simulink model "sampleModel1910"  (R2023a)
settings: Solver=VariableStepAuto  StartTime=0.0  StopTime=10.0  RelTol=1e-3
libraries: hdlsllib x3, simulink x1
settings Model: Creator=user1  LastModifiedBy=user1

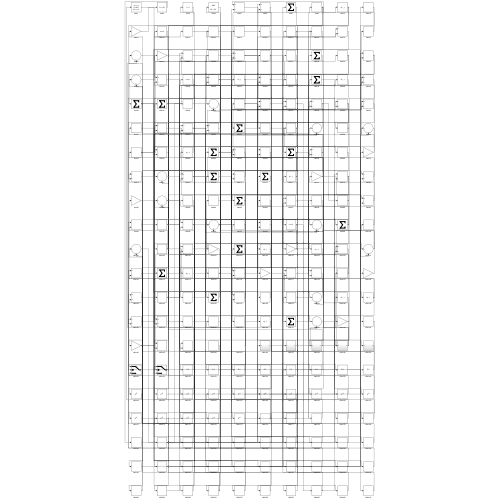
[thumbnail: Simulink's stored preview of the top-level diagram]
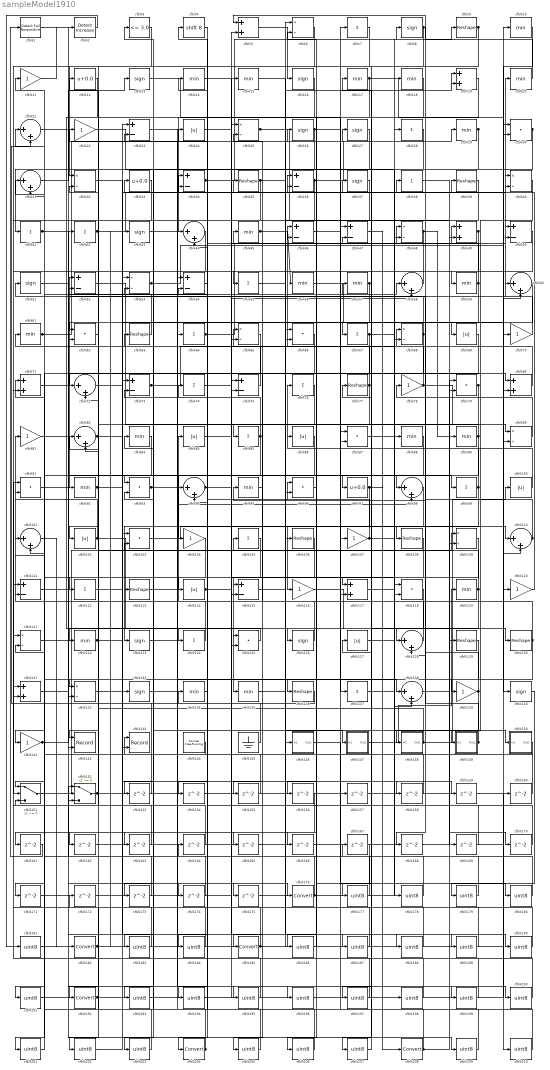
== system sampleModel1910 ==
  cfblk1 : hdlsllib/Logic and Bit Operations/Detect Fall Nonpositive  vinit=0  OutDataTypeStr=boolean
  cfblk{10,14..15,17..18,20,29,45,56..57,59,61,83,88..89,92,95,119,122,134..135} (21 alike) : MinMax
  cfblk{24,69,84,86,100,102,114,127} (8 alike) : Abs  SaturateOnIntegerOverflow=off
  cfblk{21,31,44,58,60,72,82,94,98,101,110,128,138} (13 alike) : Sum  Inputs=|++
  cfblk{30,62,66,79,87,91,93,96,103,118,125} (11 alike) : DotProduct  OutDataTypeStr=Inherit: Inherit via internal rule
  cfblk{11,22,70,78,81,104,107,116,120,139,141} (11 alike) : Gain
  cfblk{7,28,38,41..42,55,64,67,74,76,85,99,105,112,124,137} (16 alike) : Sum  Inputs=+
  cfblk{9,35,39,63,77,106,108,113,129..130,136} (11 alike) : Reshape
  cfblk{6,25,32,40,48,53,65,68,90,109,121,132} (12 alike) : Product  Inputs=*/  RndMeth=Zero  SaturateOnIntegerOverflow=on
  cfblk{23,34,36,46..47,50,52,54,73,75,111,115} (12 alike) : Sum  Inputs=+-
  cfblk{5,19,49,71,80,117,131} (7 alike) : Sum
  cfblk12 : Bias  Bias=0.0  SaturateOnIntegerOverflow=off
  cfblk{8,13,16,26..27,37,43,51,123,126,133,140} (12 alike) : Signum
  cfblk142 : Record  FileSettingsInternal="{\"entries\":[{\"content\":{\"excelSettings\":{\"content\":{},\"type\":\"Streamout.ExcelSettings\"}},\"type\":\"Streamout.FileSettingStorage\",\"uuid\":\"\"}],\"packageUris\":[\"http:\\/\\/schema.mathworks.com\\/mf0\\/streamout_blocks\\/R2020a\"],\"version\":\"1.0\"}"  Layout=[1 1]  SignalsInternal="{\"entries\":[{\"content\":{\"signals\":[{\"content\":{\"blockPath\":[],\"dimensions\":[1],\"domain\":\"\",\"lineColor\":\"#a2142f\",\"plots\":[1],\"port\":1,\"signalID\":5086,\"signalName\":\"XY Graph:1\"},\"type\":\"RecordBlkView.Signal\",\"uuid\":\"\"},{\"content\":{\"blockPath\":[],\"dimensions\":[1],\"domain\":\"\",\"lineColor\":\"#139fff\",\"plots\":[1],\"port\":2,\"signalID\":5089,\"signalName\":\"XY Graph:2\"},\"type\":\"RecordBlkView.Signal\",\"uuid\":\"\"}]},\"type\":\"RecordBlkView.InputSignals\",\"uuid\":\"\"}],\"packageUris\":[\"http:\\/\\/schema.mathworks.com\\/mf0\\/streamout_blocks\\/R2020a\"],\"version\":\"1.0\"}"  VisualizationBindings="{\"xyplotplugin\":{\"info\":[{\"series\":[{\"bindingParametersList\":[{\"parameter\":\"X-Axis\",\"signalID\":5086,\"signalName\":\"XY Graph:1\"},{\"parameter\":\"Y-Axis\",\"signalID\":5089,\"signalName\":\"XY Graph:2\"}],\"seriesID\":15448}],\"subplotID\":1}]}}"  CompatibilityTag=XY  st=-1
  cfblk143 : Record  FileSettingsInternal="{\"entries\":[{\"content\":{\"excelSettings\":{\"content\":{},\"type\":\"Streamout.ExcelSettings\"}},\"type\":\"Streamout.FileSettingStorage\",\"uuid\":\"\"}],\"packageUris\":[\"http:\\/\\/schema.mathworks.com\\/mf0\\/streamout_blocks\\/R2020a\"],\"version\":\"1.0\"}"  Layout=[1 1]  SignalsInternal="{\"entries\":[{\"content\":{\"signals\":[{\"content\":{\"blockPath\":[],\"dimensions\":[1],\"domain\":\"\",\"lineColor\":\"#a2142f\",\"plots\":[1],\"port\":1,\"signalID\":5094,\"signalName\":\"XY Graph:1\"},\"type\":\"RecordBlkView.Signal\",\"uuid\":\"\"},{\"content\":{\"blockPath\":[],\"dimensions\":[1],\"domain\":\"\",\"lineColor\":\"#139fff\",\"plots\":[1],\"port\":2,\"signalID\":5097,\"signalName\":\"XY Graph:2\"},\"type\":\"RecordBlkView.Signal\",\"uuid\":\"\"}]},\"type\":\"RecordBlkView.InputSignals\",\"uuid\":\"\"}],\"packageUris\":[\"http:\\/\\/schema.mathworks.com\\/mf0\\/streamout_blocks\\/R2020a\"],\"version\":\"1.0\"}"  VisualizationBindings="{\"xyplotplugin\":{\"info\":[{\"series\":[{\"bindingParametersList\":[{\"parameter\":\"X-Axis\",\"signalID\":5094,\"signalName\":\"XY Graph:1\"},{\"parameter\":\"Y-Axis\",\"signalID\":5097,\"signalName\":\"XY Graph:2\"}],\"seriesID\":38158}],\"subplotID\":1}]}}"  CompatibilityTag=XY  st=-1
  cfblk144 : hdlsllib/Sources/Counter Free-Running  NumBits=16  tsamp=-1
  cfblk145 : Ground
  cfblk146 : Subsystem
      settings: LibrarySourceBlock=|
      | hdlsllib/Ports &
      | Subsystems/Subsystem
  cfblk147 : Subsystem
      settings: LibrarySourceBlock=|
      | hdlsllib/Ports &
      | Subsystems/Subsystem
  cfblk148 : Subsystem
      settings: LibrarySourceBlock=|
      | hdlsllib/Ports &
      | Subsystems/Subsystem
  cfblk149 : Subsystem
      settings: LibrarySourceBlock=|
      | hdlsllib/Ports &
      | Subsystems/Subsystem
  cfblk150 : Subsystem
      settings: LibrarySourceBlock=|
      | hdlsllib/Ports &
      | Subsystems/Subsystem
  cfblk151 : Switch  SaturateOnIntegerOverflow=off  InputSameDT=off
  cfblk152 : Switch  SaturateOnIntegerOverflow=off  InputSameDT=off
  cfblk{153..175} (23 alike) : Delay  SampleTime=1
  cfblk{176,182,185,192,204,208} (6 alike) : DataTypeConversion  SaturateOnIntegerOverflow=off  RndMeth=Floor
  cfblk{177..181,183..184,186..191,193..203,205..207,209..210} (29 alike) : DataTypeConversion  OutDataTypeStr=uint8  SaturateOnIntegerOverflow=off  RndMeth=Floor
  cfblk2 : simulink/Logic and Bit Operations/Detect Increase  vinit=0.0  OutDataTypeStr=boolean
      settings: LibrarySourceBlock=|
      | hdlsllib/Logic and Bit
      | Operations/Detect
      | Increase
  cfblk3 : hdlsllib/Logic and Bit Operations/Compare To Constant  relop=<=  const=3.0  OutDataTypeStr=boolean
  cfblk33 : Bias  Bias=0.0  SaturateOnIntegerOverflow=off
  cfblk4 : ArithShift  BitShiftNumber=8
  cfblk97 : Bias  Bias=0.0  SaturateOnIntegerOverflow=off
  wires:
  cfblk65/1 -> cfblk92/1
  cfblk64/1 -> cfblk48/1, cfblk36/2
  cfblk148/1(Out1) -> cfblk100/1, cfblk52/2
  cfblk77/1 -> cfblk46/1, cfblk94/2
  cfblk120/1 -> cfblk33/1
  cfblk115/1 -> cfblk6/1
  cfblk5/1 -> cfblk16/1
  cfblk58/1 -> cfblk55/1
  cfblk16/1 -> cfblk44/1
  cfblk12/1 -> cfblk126/1
  cfblk150/1(Out1) -> cfblk84/1
  cfblk61/1 -> cfblk24/1, cfblk60/1
  cfblk48/1 -> cfblk89/1, cfblk72/1
  cfblk131/1 -> cfblk42/1
  cfblk6/1 -> cfblk32/1
  cfblk116/1 -> cfblk128/1
  cfblk128/1 -> cfblk81/1
  cfblk98/1 -> cfblk116/1
  cfblk104/1 -> cfblk114/1
  cfblk52/1 -> cfblk90/1
  cfblk99/1 -> cfblk123/1, cfblk77/1, cfblk94/1
  cfblk11/1 -> cfblk2/1
  cfblk114/1 -> cfblk74/1, cfblk188/1
  cfblk79/1 -> cfblk102/1, cfblk148/1(In1)
  cfblk50/1 -> cfblk59/1
  cfblk97/1 -> cfblk173/1, cfblk198/1
  cfblk25/1 -> cfblk107/1, cfblk19/2, cfblk49/2
  cfblk136/1 -> cfblk21/2
  cfblk151/1 -> cfblk64/1
  cfblk28/1 -> cfblk41/1
  cfblk102/1 -> cfblk130/1, cfblk71/1
  cfblk34/1 -> cfblk8/1, cfblk58/2
  cfblk113/1 -> cfblk138/1
  cfblk27/1 -> cfblk113/1
  cfblk72/1 -> cfblk133/1
  cfblk85/1 -> cfblk3/1, cfblk104/1
  cfblk70/1 -> cfblk20/1
  cfblk68/1 -> cfblk36/1, cfblk161/1
  cfblk88/1 -> cfblk141/1
  cfblk46/1 -> cfblk19/1
  cfblk45/1 -> cfblk56/1, cfblk147/1(In1)
  cfblk149/1(Out1) -> cfblk95/1, cfblk96/1
  cfblk145/1 -> cfblk12/1
  cfblk91/1 -> cfblk124/1
  cfblk71/1 -> cfblk52/1
  cfblk57/1 -> cfblk17/1, cfblk184/1
  cfblk32/1 -> cfblk69/1
  cfblk103/1 -> cfblk108/1
  cfblk112/1 -> cfblk26/1
  cfblk7/1 -> cfblk192/1
  cfblk125/1 -> cfblk122/1
  cfblk62/1 -> cfblk142/1
  cfblk60/1 -> cfblk67/1
  cfblk55/1 -> cfblk38/1
  cfblk41/1 -> cfblk80/1, cfblk99/1
  cfblk130/1 -> cfblk46/2, cfblk139/1, cfblk61/1
  cfblk78/1 -> cfblk120/1, cfblk31/2
  cfblk20/1 -> cfblk5/1
  cfblk94/1 -> cfblk50/1, cfblk49/1
  cfblk69/1 -> cfblk136/1
  cfblk133/1 -> cfblk27/1
  cfblk80/1 -> cfblk45/1
  cfblk105/1 -> cfblk135/1
  cfblk13/1 -> cfblk137/1
  cfblk66/1 -> cfblk132/1
  cfblk47/1 -> cfblk208/1
  cfblk29/1 -> cfblk128/2, cfblk166/1
  cfblk14/1 -> cfblk176/1
  cfblk110/1 -> cfblk51/1, cfblk65/1
  cfblk82/1 -> cfblk40/2, cfblk174/1
  cfblk59/1 -> cfblk22/1, cfblk62/2
  cfblk86/1 -> cfblk185/1
  cfblk40/1 -> cfblk149/1(In1)
  cfblk129/1 -> cfblk151/1
  cfblk22/1 -> cfblk118/1
  cfblk89/1 -> cfblk85/1, cfblk96/2
  cfblk109/1 -> cfblk115/1
  cfblk119/1 -> cfblk25/2, cfblk82/1, cfblk197/1
  cfblk56/1 -> cfblk140/1
  cfblk54/1 -> cfblk34/1
  cfblk37/1 -> cfblk112/1
  cfblk67/1 -> cfblk37/1, cfblk138/2, cfblk165/1, cfblk171/1
  cfblk93/1 -> cfblk98/2, cfblk153/1
  cfblk53/1 -> cfblk10/1, cfblk125/1
  cfblk10/1 -> cfblk90/2
  cfblk152/1 -> cfblk75/2, cfblk82/2
  cfblk35/1 -> cfblk106/1, cfblk115/2
  cfblk81/1 -> cfblk142/2
  cfblk73/1 -> cfblk28/1, cfblk98/1
  cfblk124/1 -> cfblk73/2
  cfblk3/1 -> cfblk131/2
  cfblk26/1 -> cfblk110/1, cfblk72/2
  cfblk135/1 -> cfblk50/2
  cfblk92/1 -> cfblk54/2, cfblk189/1
  cfblk122/1 -> cfblk109/1, cfblk35/1
  cfblk141/1 -> cfblk58/1, cfblk175/1
  cfblk84/1 -> cfblk5/2
  cfblk24/1 -> cfblk118/2
  cfblk63/1 -> cfblk31/1
  cfblk31/1 -> cfblk13/1
  cfblk42/1 -> cfblk40/1, cfblk65/2
  cfblk90/1 -> cfblk78/1
  cfblk75/1 -> cfblk44/2
  cfblk17/1 -> cfblk110/2, cfblk132/2
  cfblk74/1 -> cfblk97/1
  cfblk117/1 -> cfblk29/1
  cfblk9/1 -> cfblk62/1, cfblk154/1
  cfblk30/1 -> cfblk68/2, cfblk193/1
  cfblk87/1 -> cfblk150/1(In1)
  cfblk107/1 -> cfblk53/2, cfblk39/1
  cfblk83/1 -> cfblk93/1
  cfblk100/1 -> cfblk76/1
  cfblk101/1 -> cfblk182/1
  cfblk39/1 -> cfblk152/2
  cfblk139/1 -> cfblk68/1, cfblk183/1
  cfblk137/1 -> cfblk9/1
  cfblk134/1 -> cfblk204/1
  cfblk144/1 -> cfblk143/1
  cfblk49/1 -> cfblk152/3, cfblk151/2
  cfblk147/1(Out1) -> cfblk119/1
  cfblk33/1 -> cfblk143/2
  cfblk36/1 -> cfblk18/1, cfblk71/2
  cfblk126/1 -> cfblk105/1
  cfblk123/1 -> cfblk57/1
  cfblk8/1 -> cfblk117/1, cfblk168/1, cfblk207/1
  cfblk153/1 -> cfblk73/1
  cfblk154/1 -> cfblk80/2
  cfblk95/1 -> cfblk155/1
  cfblk155/1 -> cfblk53/1
  cfblk19/1 -> cfblk156/1
  cfblk157/1 -> cfblk109/2
  cfblk43/1 -> cfblk158/1
  cfblk158/1 -> cfblk6/2
  cfblk132/1 -> cfblk159/1
  cfblk160/1 -> cfblk91/2
  cfblk161/1 -> cfblk1/1
  cfblk18/1 -> cfblk162/1
  cfblk162/1 -> cfblk48/2
  cfblk44/1 -> cfblk163/1
  cfblk163/1 -> cfblk131/1
  cfblk164/1 -> cfblk32/2
  cfblk165/1 -> cfblk79/2
  cfblk166/1 -> cfblk117/2
  cfblk168/1 -> cfblk60/2
  cfblk38/1 -> cfblk169/1
  cfblk169/1 -> cfblk34/2
  cfblk138/1 -> cfblk170/1
  cfblk170/1 -> cfblk25/1
  cfblk171/1 -> cfblk125/2
  cfblk173/1 -> cfblk21/1
  cfblk174/1 -> cfblk152/1
  cfblk175/1 -> cfblk88/1
  cfblk176/1 -> cfblk164/1, cfblk75/1
  cfblk118/1 -> cfblk177/1
  cfblk177/1 -> cfblk14/1
  cfblk127/1 -> cfblk178/1
  cfblk178/1 -> cfblk83/1
  cfblk140/1 -> cfblk179/1
  cfblk179/1 -> cfblk127/1
  cfblk146/1(Out1) -> cfblk180/1
  cfblk180/1 -> cfblk93/2
  cfblk2/1 -> cfblk181/1
  cfblk181/1 -> cfblk146/1(In1)
  cfblk182/1 -> cfblk160/1, cfblk157/1, cfblk66/2, cfblk43/1
  cfblk183/1 -> cfblk101/1
  cfblk184/1 -> cfblk101/2
  cfblk185/1 -> cfblk11/1, cfblk79/1
  cfblk96/1 -> cfblk186/1
  cfblk186/1 -> cfblk86/1
  cfblk121/1 -> cfblk187/1
  cfblk187/1 -> cfblk66/1
  cfblk188/1 -> cfblk121/1
  cfblk189/1 -> cfblk121/2
  cfblk15/1 -> cfblk190/1
  cfblk190/1 -> cfblk87/1
  cfblk106/1 -> cfblk191/1
  cfblk191/1 -> cfblk15/1
  cfblk192/1 -> cfblk87/2, cfblk70/1
  cfblk193/1 -> cfblk7/1
  cfblk4/1 -> cfblk194/1
  cfblk194/1 -> cfblk30/2
  cfblk51/1 -> cfblk195/1
  cfblk195/1 -> cfblk4/1
  cfblk23/1 -> cfblk196/1
  cfblk196/1 -> cfblk30/1
  cfblk197/1 -> cfblk23/1
  cfblk198/1 -> cfblk23/2
  cfblk111/1 -> cfblk199/1
  cfblk199/1 -> cfblk91/1
  cfblk1/1 -> cfblk200/1
  cfblk200/1 -> cfblk111/1
  cfblk156/1 -> cfblk201/1
  cfblk201/1 -> cfblk111/2
  cfblk172/1 -> cfblk202/1
  cfblk202/1 -> cfblk103/1
  cfblk108/1 -> cfblk203/1
  cfblk203/1 -> cfblk172/1
  cfblk204/1 -> cfblk54/1, cfblk103/2
  cfblk76/1 -> cfblk205/1
  cfblk205/1 -> cfblk134/1
  cfblk167/1 -> cfblk206/1
  cfblk206/1 -> cfblk151/3
  cfblk207/1 -> cfblk167/1
  cfblk208/1 -> cfblk129/1, cfblk63/1
  cfblk21/1 -> cfblk209/1
  cfblk209/1 -> cfblk47/1
  cfblk159/1 -> cfblk210/1
  cfblk210/1 -> cfblk47/2

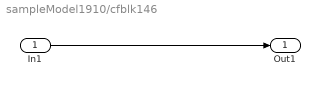
== system sampleModel1910/cfblk146 ==
  In1 : Inport
  Out1 : Outport
  wires:
  In1/1 -> Out1/1

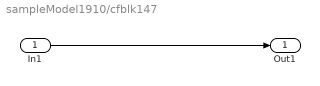
== system sampleModel1910/cfblk147 ==
  In1 : Inport
  Out1 : Outport
  wires:
  In1/1 -> Out1/1

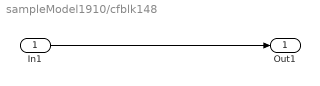
== system sampleModel1910/cfblk148 ==
  In1 : Inport
  Out1 : Outport
  wires:
  In1/1 -> Out1/1

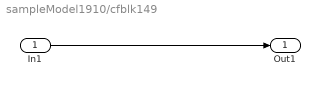
== system sampleModel1910/cfblk149 ==
  In1 : Inport
  Out1 : Outport
  wires:
  In1/1 -> Out1/1

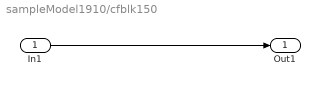
== system sampleModel1910/cfblk150 ==
  In1 : Inport
  Out1 : Outport
  wires:
  In1/1 -> Out1/1
